simulink model "ARCH_AT2_artificial"  (R2019b)
settings: Solver=FixedStepAuto  StartTime=0.0  StopTime=10.0  FixedStep=fixedStepSize  RelTol=1e-3
undefined symbols (not defined in the file): ARCH_AT2_rpmLimit, ARCH_AT2_rpmLimitAct, artificial_ARCH_AT2_constant
settings Model: Creator=JEDDELAN  LastModifiedBy=JEDDELAN
settings DataIOCC: SaveOutput=off  SaveTime=off  ReturnWorkspaceOutputs=off
settings DebuggingCC: ArithmeticOperatorsInVariantConditions=warning
settings SFSimCC: SimUseLocalCustomCode=off  CustomCodeUndefinedFunction=UseInterfaceOnly
settings RTWCC: RTWUseLocalCustomCode=off
settings GRTTargetCC: CombineOutputUpdateFcns=off  MatFileLogging=off

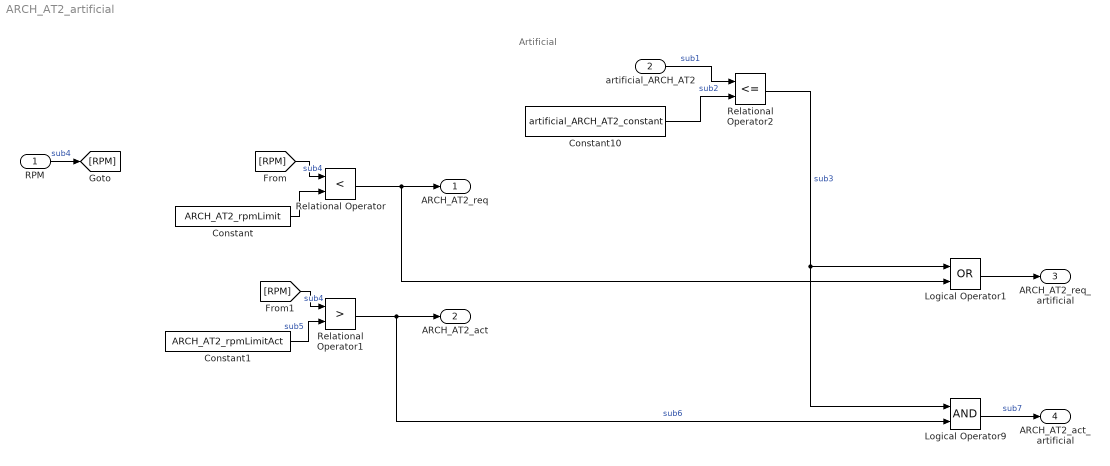
== system ARCH_AT2_artificial ==
  note: Artificial
  RPM : Inport
  artificial_ARCH_AT2 : Inport  Port=2
  Constant : Constant  Value=ARCH_AT2_rpmLimit
  Constant1 : Constant  Value=ARCH_AT2_rpmLimitAct
  Constant10 : Constant  Value=artificial_ARCH_AT2_constant
  Logical Operator1 : Logic  Operator=OR  AllPortsSameDT=off  OutDataTypeStr=boolean
  Logical Operator9 : Logic  AllPortsSameDT=off  OutDataTypeStr=boolean
  Relational Operator : RelationalOperator  Operator=<  OutDataTypeStr=boolean  RndMeth=Simplest
  Relational Operator1 : RelationalOperator  Operator=>  OutDataTypeStr=boolean  RndMeth=Simplest
  Relational Operator2 : RelationalOperator  Operator=<=  OutDataTypeStr=boolean  RndMeth=Simplest
  ARCH_AT2_req : Outport  OutDataTypeStr=boolean  PortDimensions=1  VectorParamsAs1DForOutWhenUnconnected=off
  ARCH_AT2_act : Outport  Port=2  OutDataTypeStr=boolean  PortDimensions=1  VectorParamsAs1DForOutWhenUnconnected=off
  ARCH_AT2_req_artificial : Outport  Port=3  OutDataTypeStr=boolean  PortDimensions=1  VectorParamsAs1DForOutWhenUnconnected=off
  ARCH_AT2_act_artificial : Outport  Port=4  OutDataTypeStr=boolean  PortDimensions=1  VectorParamsAs1DForOutWhenUnconnected=off
  wires:
  RPM/1 -> [RPM]  "sub4"
  Constant/1 -> Relational Operator/2
  [RPM] -> Relational Operator/1  "sub4"
  Constant1/1 -> Relational Operator1/2  "sub5"
  [RPM] -> Relational Operator1/1  "sub4"
  Relational Operator1/1 -> Logical Operator9/2, ARCH_AT2_act/1  "sub6"
  Relational Operator/1 -> Logical Operator1/2, ARCH_AT2_req/1
  artificial_ARCH_AT2/1 -> Relational Operator2/1  "sub1"
  Logical Operator1/1 -> ARCH_AT2_req_artificial/1
  Relational Operator2/1 -> Logical Operator9/1, Logical Operator1/1  "sub3"
  Logical Operator9/1 -> ARCH_AT2_act_artificial/1  "sub7"
  Constant10/1 -> Relational Operator2/2  "sub2"
